simulink model "PMSM_temperature_estimation_EKF"  (R2023b)
settings: Solver=VariableStepAuto  StartTime=0.0  StopTime=10  FixedStep=dt  RelTol=1e-3  AbsTol=1e-3
values from neighbouring files (symbols this model uses):
  CF_fc = 1/(20*Ts)    (= 5)    [controller_parameters.m]
  CF_k = 1    [controller_parameters.m]
  dt = 50e-6    (= 5e-05)    [config.m]
  dt_speed_control = 0.001    [config.m]
  max_power = 50e3    (= 50000)    [config.m]
  max_torque = 220    [config.m]
  N = 6    [config.m]
  ratio_rotor = 0.75    [config.m]
  Rd_percent_rotor = ratio_rotor*100    (= 75)    [config.m]
  Rm_percent_rotor = ratio_rotor*100    (= 75)    [config.m]
  rotor_initial_temperatures = 298.15    [config.m]
  stator_initial_temperatures = [298.15;298.15;298.15]    [config.m]
  stator_thermal_mass = 100    [config.m]
  Ts = 0.01    [controller_parameters.m]
undefined symbols (not defined in the file or in its folder): cex, ch, cJ, DiscIntNeverNeededParam
libraries: fl_lib x152, nesl_utility x45, fl_ps_legacy_lib x3, sharedTrackingLibrary x1, ee_lib x1, SignalEditorBlockLib x1, simulink x1
(part 1 of 3)
Description:
  | PMSM with Thermal Model
settings Model: Creator=The MathWorks, Inc.  LastModifiedBy=block
settings SolverCC: AutoScaleAbsTol=off  AlgebraicLoopSolver=TrustRegion
settings DataIOCC: MaxDataPoints=210000  SaveFormat=Array  ReturnWorkspaceOutputsName=simOut
settings OptimizationCC: BlockReduction=off  BooleanDataType=off  LifeSpan=inf
settings DebuggingCC: SaveWithParameterizedLinksMsg=none  UnderspecifiedInitializationDetection=Classic  MergeDetectMultiDrivingBlocksExec=none  SignalResolutionControl=TryResolveAllWithWarning  UnconnectedInputMsg=warning  UnconnectedOutputMsg=warning  UnconnectedLineMsg=warning  AllowSymbolicDim=off  SFUnexpectedBacktrackingDiag=warning  SFNoUnconditionalDefaultTransitionDiag=warning  SFExecutionAtInitializationDiag=none  ArithmeticOperatorsInVariantConditions=warning
settings HardwareCC: ProdBitPerPointer=32  ProdBitPerSizeT=32  ProdBitPerPtrDiffT=32  ProdLargestAtomicFloat=None  ProdIntDivRoundTo=Undefined  ProdEndianess=Unspecified  ProdWordSize=32  ProdHWDeviceType=32-bit Generic  TargetUnknown=on
settings ModelReferenceCC: EnableRefExpFcnMdlSchedulingChecks=on  PropagateSignalLabelsOutOfModel=off
settings SFSimCC: SimUseLocalCustomCode=off  CustomCodeUndefinedFunction=UseInterfaceOnly
settings RTWCC: RTWUseLocalCustomCode=off  DLArmComputeVersion=19.05
settings CodeAppCC: StateflowObjectComments=on
settings GRTTargetCC: TargetLangStandard=C89/C90 (ANSI)
settings ConfigComp: CovMetricSettings=dw  CovSaveCumulativeToWorkspaceVar=on  CovSaveSingleToWorkspaceVar=on  CovExternalEMLEnable=off  CovSFcnEnable=off
settings SimscapeCC: SimscapeLogType=all  SimscapeLogSimulationStatistics=on  SimscapeLogName=simlog_PMSMWithThermal  SimscapeLogDecimation=10  SimscapeLogDataHistory=210000

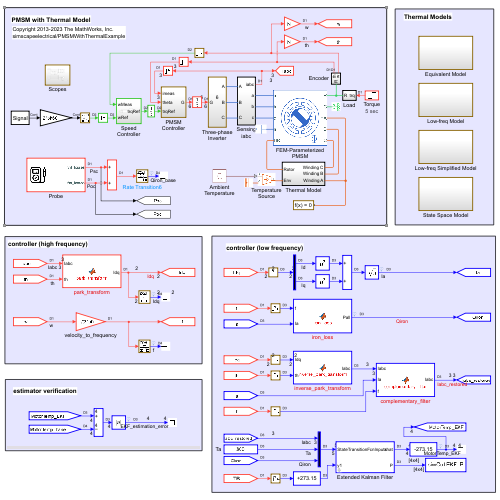
[thumbnail: Simulink's stored preview of the top-level diagram]
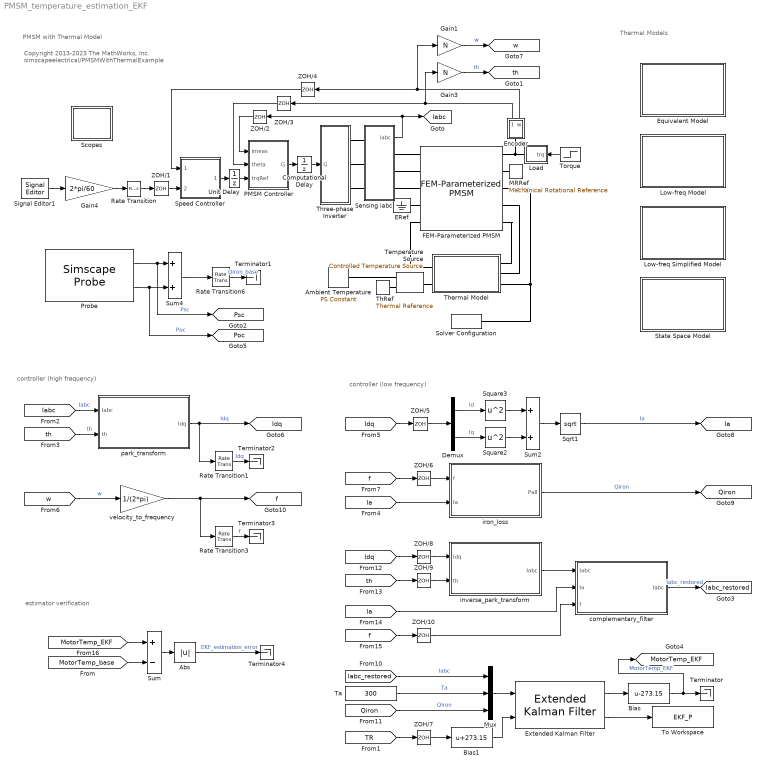
== system PMSM_temperature_estimation_EKF ==
  note: PMSM with Thermal Model
  note: controller (high frequency)
  note: controller (low frequency)
  note: Copyright 2013-2023 The MathWorks, Inc.
      | simscapeelectrical/PMSMWithThermalExample
  note: Thermal Models
  note: estimator verification
  Abs : Abs  SaturateOnIntegerOverflow=off
  Ambient Temperature : fl_lib/Physical Signals/Sources/PS Constant  constant=300
  Bias : Bias  Bias=-273.15  SaturateOnIntegerOverflow=off
  Bias1 : Bias  Bias=273.15  SaturateOnIntegerOverflow=off
  Computational Delay : UnitDelay  SampleTime=dt  HasFrameUpgradeWarning=on
  Demux : Demux  Outputs=2
  ERef : fl_lib/Electrical/Electrical Elements/Electrical Reference
  Encoder : Subsystem
  Equivalent Model : Subsystem  Tag=PublishSubsystem
  Extended Kalman Filter : sharedTrackingLibrary/Extended Kalman Filter  StateTransitionFcn=state_equation_discrete  HasStateTransitionJacobianFcn=off  HasAdditiveProcessNoise=Additive  ProcessNoise=EKF_Q  HasTimeVaryingProcessNoise=off  HasStateTransitionFcnExtraArgument=1  InitialState=EKF_x0  InitialStateCovariance=EKF_P0  MeasurementFcn1=output_equation  HasMeasurementJacobianFcn1=off  HasMeasurementEnablePort1=off  HasAdditiveMeasurementNoise1=Additive  MeasurementNoise1=EKF_R  HasTimeVaryingMeasurementNoise1=off  HasMeasurementFcnExtraArgument1=0  HasMeasurementWrapping1=off  MeasurementFcn2=myMeasurementFcn  HasMeasurementJacobianFcn2=off  HasMeasurementEnablePort2=off  HasAdditiveMeasurementNoise2=Additive  MeasurementNoise2=1  HasTimeVaryingMeasurementNoise2=off  HasMeasurementFcnExtraArgument2=0  HasMeasurementWrapping2=off  MeasurementFcn3=myMeasurementFcn  HasMeasurementJacobianFcn3=off  HasMeasurementEnablePort3=off  HasAdditiveMeasurementNoise3=Additive  MeasurementNoise3=1  HasTimeVaryingMeasurementNoise3=off  HasMeasurementFcnExtraArgument3=0  HasMeasurementWrapping3=off  MeasurementFcn4=myMeasurementFcn  HasMeasurementJacobianFcn4=off  HasMeasurementEnablePort4=off  HasAdditiveMeasurementNoise4=Additive  MeasurementNoise4=1  HasTimeVaryingMeasurementNoise4=off  HasMeasurementFcnExtraArgument4=0  HasMeasurementWrapping4=off  MeasurementFcn5=myMeasurementFcn  HasMeasurementJacobianFcn5=off  HasMeasurementEnablePort5=off  HasAdditiveMeasurementNoise5=Additive  MeasurementNoise5=1  HasTimeVaryingMeasurementNoise5=off  HasMeasurementFcnExtraArgument5=0  HasMeasurementWrapping5=off  EnableMultirate=off  StateTransitionFcnSampleTime=1  MeasurementFcn1SampleTime=1  MeasurementFcn2SampleTime=1  MeasurementFcn3SampleTime=1  MeasurementFcn4SampleTime=1  MeasurementFcn5SampleTime=1  UseCurrentEstimator=on  OutputStateCovariance=on  DataType=double  SampleTime=Ts  NumberOfMeasurements=1
  FEM-Parameterized PMSM : ee_lib/Electromechanical/Permanent Magnet/FEM-Parameterized PMSM  parameterization=1  winding_type=ee.enum.statorconnection.wye  iVec=iVec_th A  xVec=xVec_th deg  dfluxdiMatrix=dfluxdiMatrix Wb/A  dfluxdxMatrix=dfluxdxMatrix Wb/rad  calculate_torque_matrix=1  TorqueMatrix=[0, 0.3, - 0.3, 0; 0, 0, 0, 0; 0, - 0.3, 0.3, 0] N*m  idVec1=[-200.0, 0.0, 200.0] A  iqVec1=[-200.0, 0.0, 200.0] A  LdMatrix=0.0002 * ones(3, 3) H  LqMatrix=0.0002 * ones(3, 3) H  PmMatrix=0.1 * ones(3, 3) Wb  N=6  interp_method=1  Rs=Rs Ohm  Ms=Ms H  L0=0.00016 H  loss_param=ee.enum.fem_motor.ironLossesExtended.empirical  losses_oc=losses_oc W  losses_sc=losses_sc W  f_losses=f_losses Hz  Isc_losses=Isc_losses A  Inertia=0.02 kg*m^2  lam=0 N*m/(rad/s)  i_d_specify=off  i_d_priority=None  i_d=0 A  i_d_nominal_specify=off  i_d_nominal_unit=A  i_d_nominal_value=1  i_q_specify=off  i_q_priority=None  i_q=0 A  i_q_nominal_specify=off  i_q_nominal_unit=A  i_q_nominal_value=1  torque_specify=off  torque_priority=None  torque=0 N*m  torque_nominal_specify=off  torque_nominal_unit=N*m  torque_nominal_value=1  angular_velocity_specify=on  angular_velocity_priority=High  angular_velocity=0 rpm  angular_velocity_nominal_specify=off  angular_velocity_nominal_unit=rpm  angular_velocity_nominal_value=1  angular_position_specify=on  angular_position_priority=High  angular_position=0 deg  angular_position_nominal_specify=off  angular_position_nominal_unit=deg  angular_position_nominal_value=1  Tmeas=Tmeas K  alpha=alpha 1/K  alpha_flux=alpha_flux 1/K  stator_thermal_mass=stator_thermal_mass J/K  stator_initial_temperatures=stator_initial_temperatures K  rotor_thermal_mass=rotor_thermal_mass J/K  rotor_initial_temperature=rotor_initial_temperatures K  Rm_percent_rotor=Rm_percent_rotor  Rd_percent_rotor=Rm_percent_rotor  idVec=[-200, 0, 200] A  iqVec=[-200, 0, 200] A  dfluxAdiaMatrix3D=zeros(3, 3, 4) Wb/A  dfluxAdibMatrix3D=zeros(3, 3, 4) Wb/A  dfluxAdicMatrix3D=zeros(3, 3, 4) Wb/A  dfluxAdxMatrix3D=zeros(3, 3, 4) Wb/rad  TorqueMatrix3D=zeros(3, 3, 4) N*m  iaVec=[-200, 0, 200] A  ibVec=[-200, 0, 200] A  icVec=[-200, 0, 200] A  dfluxAdiaMatrix=zeros(3, 3, 3, 4) Wb/A  dfluxAdibMatrix=zeros(3, 3, 3, 4) Wb/A  dfluxAdicMatrix=zeros(3, 3, 3, 4) Wb/A  dfluxAdxMatrix=zeros(3, 3, 3, 4) Wb/rad  param_dq0=ee.enum.fem_motor.fluxTabulationOption.DQcartesian  winding_type_dq0=ee.enum.statorconnection.wye  expose_neutral_port=ee.enum.fem_motor.exposeNeutralPort.no  nPolePairs=4  parks_type=ee.enum.fem_motor.parksType.QleadsD_AphaseToDaxis  idVec2=[-200, 0, 200] A  iqVec2=[-200, 0, 200] A  magVec2=[0, 100, 200] A  betaVec2=[-180, -90, 0, 90, 180] deg  xVec2=[0, 15, 30, 45, 60, 75, 90] deg  fluxD_dq0=zeros(3, 3, 7) Wb  fluxQ_dq0=zeros(3, 3, 7) Wb  fluxA_dq0=zeros(3, 3, 7) Wb  Torque_dq0=ones(3, 3, 7) N*m  fluxD_IBX=zeros(3, 5, 7) Wb  fluxQ_IBX=zeros(3, 5, 7) Wb  fluxA_IBX=zeros(3, 5, 7) Wb  Torque_IBX=zeros(3, 5, 7) N*m  rotorLossCoeff_k_h_DQ=zeros(3, 3) W/Hz  rotorLossCoeff_k_J_DQ=zeros(3, 3) W/Hz^2  rotorLossCoeff_k_ex_DQ=zeros(3, 3) W/Hz^(3/2)  rotorLossCoeff_k_h_IB=zeros(3, 5) W/Hz  rotorLossCoeff_k_J_IB=zeros(3, 5) W/Hz^2  rotorLossCoeff_k_ex_IB=zeros(3, 5) W/Hz^(3/2)  statorLossCoeff_k_h_DQ=zeros(3, 3) W/Hz  statorLossCoeff_k_J_DQ=zeros(3, 3) W/Hz^2  statorLossCoeff_k_ex_DQ=zeros(3, 3) W/Hz^(3/2)  statorLossCoeff_k_h_IB=zeros(3, 5) W/Hz  statorLossCoeff_k_J_IB=zeros(3, 5) W/Hz^2  statorLossCoeff_k_ex_IB=zeros(3, 5) W/Hz^(3/2)  wVec=[1000, 2000] rpm  rotorLossTable_DQ=zeros(3, 3, 2) W  rotorLossTable_IB=zeros(3, 5, 2) W  statorLossTable_DQ=zeros(3, 3, 2) W  statorLossTable_IB=zeros(3, 5, 2) W  electrical_torque_before_iron_losses_specify=off  electrical_torque_before_iron_losses_priority=None  electrical_torque_before_iron_losses=0 N*m  electrical_torque_before_iron_losses_nominal_specify=off  electrical_torque_before_iron_losses_nominal_unit=N*m  electrical_torque_before_iron_losses_nominal_value=1  Qrotor_specify=off  Qrotor_priority=None  Qrotor=0 J/s  Qrotor_nominal_specify=off  Qrotor_nominal_unit=J/s  Qrotor_nominal_value=1  Qstator_specify=off  Qstator_priority=None  Qstator=0 J/s  Qstator_nominal_specify=off  Qstator_nominal_unit=J/s  Qstator_nominal_value=1
      settings: InternalSimscapePortConfiguration="{\"Bottom\":[],\"Left\":[{\"id\":\"a\",\"label\":\"a\",\"type\":\"foundation.electrical.electrical\"},{\"id\":\"b\",\"label\":\"b\",\"type\":\"foundation.electrical.electrical\"},{\"id\":\"c\",\"label\":\"c\",\"type\":\"foundation.electrical.electrical\"},{\"id\":\"n\",\"label\":\"n\",\"type\":\"foundation.electrical.electrical\"},{\"id\":\"HR\",\"label\":\"HR\",\"type\":\"foundation.thermal.thermal\"}],\"Right\":[{\"id\":\"R\",\"label\":\"R\",\"type\":\"foundation.mechanical.rotational.rotational\"},{\"id\":\"C\",\"label\":\"C\",\"type\":\"foundation.mechanical.rotational.rotational\"},{\"id\":\"HA\",\"label\":\"HA\",\"type\":\"foundation.thermal.thermal\"},{\"id\":\"HB\",\"label\":\"HB\",\"type\":\"foundation.thermal.thermal\"},{\"id\":\"HC\",\"label\":\"HC\",\"type\":\"foundation.thermal.thermal\"}],\"Top\":[]}"
  Gain1 : Gain  Gain=N
  Gain3 : Gain  Gain=N
  Gain4 : Gain  Gain=2*pi/60
  Load : Subsystem
  Low-freq Model : Subsystem  Tag=PublishSubsystem
  Low-freq Simplified Model : Subsystem  Tag=PublishSubsystem
  MRRef : fl_lib/Mechanical/Rotational Elements/Mechanical Rotational Reference
  Mux : Mux  Inputs=3
  PMSM Controller : Subsystem
  Probe : SimscapeProbe  BoundBlock=1888  Variables={Vd_losses, Vm_losses}
  Rate Transition : RateTransition
  Rate Transition1 : RateTransition  OutPortSampleTime=dt_display
  Rate Transition3 : RateTransition  OutPortSampleTime=dt_display
  Rate Transition6 : RateTransition  OutPortSampleTime=dt_display
  Scopes : Subsystem
  Sensing iabc : Subsystem
  Signal Editor1 : SignalEditorBlockLib/Signal Editor  FileName=target_speed.mat  ActiveScenario=Scenario  ActiveSignal=Signal  IsBus=off  OutputBusObjectStr=Bus: BusObject  SampleTime=0  Interpolate=off  ZeroCross=off  OutputAfterFinalValue=Setting to zero  Unit=inherit  PreserveSignalName=on  ApplySigPropsToAllScenarios=on  ApplySigPropsToAllSignals=off
  Solver Configuration : nesl_utility/Solver Configuration  PhysicalDomain=network_engine_domain  SubClassName=solver  LeftPortType=input  RightPortType=generic  Tones=[]  Harmonics=[]  SimulateNoise=off  Profile=off  UseLocalSampling=off  EnableSwitchedLinearOptims=on  FrequencyDomain=off  UseCCode=off  RelTol=0.001  AbsTol=1e-06  MinStep=1e-09  ToWorkspace=off  RevertToSquareIcSolve=off  NumHomotopyIterations=100  PhasorMode=off  PhasorModeNumHarmonics=1  ConsistencySolver=NEWTON_FTOL  IndexReductionMethod=DerivativeReplacement  DoDC=off  ResidualTolerance=1e-9  ConsistencyTolSource=GLOBAL  ConsistencyAbsTol=0.001  ConsistencyRelTol=0.001  ConsistencyTolFactor=0.001  UseLocalSolver=on  LocalSolverChoice=NE_BACKWARD_EULER_ADVANCER  ResolveIndetEquations=on  FunctionEvalNumThread=1  LocalSolverSampleTime=dt  DoFixedCost=on  MaxNonlinIter=3  MaxModeIter=2  ComputeImpulses=off  ImpulseIterations=2  LinearAlgebra=auto  LinearAlgebraNumThread=0  EquationFormulation=NE_TIME_EF  DelaysMemoryBudget=1024  AutomaticFiltering=on  FilteringTimeConstant=0.001  PartitionStorageMethod=AS_NEEDED  PartitionMemoryBudget=1024  PartitionMethod=FAST  MultibodyUseLocalSolver=off  MultibodyLocalSolverChoice=ODE1  MultibodyLocalSolverSampleTime=0.001
  Speed Controller : Subsystem
  Sqrt1 : Sqrt
  Square2 : Math  Operator=square
  Square3 : Math  Operator=square
  State Space Model : Subsystem  Tag=PublishSubsystem
  Sum : Sum  Inputs=+-
  Sum2 : Sum
  Sum4 : Sum
  Ta : Constant  Value=300  SampleTime=Ts
  Temperature Source : fl_lib/Thermal/Thermal Sources/Controlled Temperature Source
  Terminator{,1..4} (5 alike) : Terminator
  ThRef : fl_lib/Thermal/Thermal Elements/Thermal Reference
  Thermal Model : Subsystem  Tag=PublishSubsystem
  Three-phase Inverter : Subsystem  VariantControl=Variant
  To Workspace : ToWorkspace  VariableName=EKF_P  SampleTime=-1
      settings: MaxDataPoints=1
  Torque : Step  Time=5  After=100  SampleTime=dt
      settings: AttributesFormatString=%<Time> sec
  Unit Delay : UnitDelay  SampleTime=dt_speed_control  HasFrameUpgradeWarning=on
  ZOH/1 : ZeroOrderHold  SampleTime=dt_speed_control
  ZOH/{5..10} (6 alike) : ZeroOrderHold  SampleTime=Ts
  ZOH/2 : ZeroOrderHold  SampleTime=dt
  ZOH/3 : ZeroOrderHold  SampleTime=dt
  ZOH/4 : ZeroOrderHold  SampleTime=dt_speed_control
  complementary_filter : MATLAB Function  TreatAsAtomicUnit=on
  inverse_park_transform : MATLAB Function  TreatAsAtomicUnit=on
  iron_loss : MATLAB Function  TreatAsAtomicUnit=on
  park_transform : MATLAB Function  TreatAsAtomicUnit=on
  velocity_to_frequency : Gain  Gain=1/(2*pi)
  tag scope: Ia=global, Iabc=global, Iabc_restored=global, Idq=global, MotorTemp_EKF=global, Poc=global, Psc=global, Qiron=global, f=global, th=global, w=global
  wires:
  Encoder/2(w) -> ZOH/4/1, Gain1/1
  ZOH/4/1 -> Speed Controller/1(wMeas)
  Speed Controller/1(trqRef) -> Unit Delay/1
  ZOH/1/1 -> Speed Controller/2(wRef)
  ZOH/3/1 -> PMSM Controller/2(theta)
  ZOH/2/1 -> PMSM Controller/1(imeas)
  PMSM Controller/1(G) -> Computational Delay/1
  Unit Delay/1 -> PMSM Controller/3(trqRef)
  Encoder/1(th) -> ZOH/3/1, Gain3/1
  Computational Delay/1 -> Three-phase Inverter/1(G)
  Sensing iabc/1(iabc) -> [Iabc], ZOH/2/1
  Torque/1 -> Load/1(trq)
  Rate Transition/1 -> ZOH/1/1
  Signal Editor1/1 -> Gain4/1
  [Iabc] -> park_transform/1(Iabc)  "Iabc"
  [th] -> park_transform/2(th)  "th"
  Probe/1 -> [Psc], Sum4/1  "Psc"
  Gain1/1 -> [w]  "w"
  Gain3/1 -> [th]  "th"
  park_transform/1(Idq) -> [Idq], Rate Transition1/1  "Idq"
  Gain4/1 -> Rate Transition/1
  ZOH/5/1 -> Demux/1
  Demux/2 -> Square2/1  "Iq"
  Demux/1 -> Square3/1  "Id"
  Square3/1 -> Sum2/1
  Square2/1 -> Sum2/2
  Sum2/1 -> Sqrt1/1
  Sqrt1/1 -> [Ia]  "Ia"
  iron_loss/1(Pall) -> [Qiron]  "Qiron"
  [f] -> ZOH/6/1
  Rate Transition6/1 -> Terminator1/1  "Qiron_base"
  Rate Transition1/1 -> Terminator2/1  "Idq"
  [Idq] -> ZOH/5/1
  [w] -> velocity_to_frequency/1  "w"
  velocity_to_frequency/1 -> [f], Rate Transition3/1
  Rate Transition3/1 -> Terminator3/1  "f"
  Sum4/1 -> Rate Transition6/1
  ZOH/6/1 -> iron_loss/1(f)
  [Ia] -> iron_loss/2(Ia)
  Probe/2 -> [Poc], Sum4/2  "Poc"
  Ta/1 -> Mux/2  "Ta"
  [Iabc_restored] -> Mux/1  "Iabc"
  [Qiron] -> Mux/3  "Qiron"
  [TR] -> ZOH/7/1
  Mux/1 -> Extended Kalman Filter/1
  ZOH/7/1 -> Bias1/1
  Bias/1 -> [MotorTemp_EKF], Terminator/1  "MotorTemp_EKF"
  Extended Kalman Filter/1 -> Bias/1
  Bias1/1 -> Extended Kalman Filter/2
  [Idq] -> ZOH/8/1
  ZOH/8/1 -> inverse_park_transform/1(Idq)
  ZOH/9/1 -> inverse_park_transform/2(th)
  [th] -> ZOH/9/1
  inverse_park_transform/1(Iabc) -> complementary_filter/1("Iabc ")
  [Ia] -> complementary_filter/2(Ia)
  [f] -> ZOH/10/1
  ZOH/10/1 -> complementary_filter/3(f)
  complementary_filter/1(Iabc) -> [Iabc_restored]  "Iabc_restored"
  Extended Kalman Filter/2 -> To Workspace/1
  [MotorTemp_EKF] -> Sum/1
  [MotorTemp_base] -> Sum/2
  Abs/1 -> Terminator4/1  "EKF_estimation_error"
  Sum/1 -> Abs/1
  connections:
  FEM-Parameterized PMSM/LConn4 -- ERef/LConn1
  FEM-Parameterized PMSM/RConn4 -- Thermal Model/RConn2
  FEM-Parameterized PMSM/RConn5 -- Thermal Model/RConn1
  FEM-Parameterized PMSM/RConn3 -- Solver Configuration/RConn1 -- Thermal Model/RConn3
  MRRef/LConn1 -- FEM-Parameterized PMSM/RConn2
  FEM-Parameterized PMSM/RConn1 -- Encoder/LConn1 -- Load/RConn1
  Three-phase Inverter/RConn1 -- Sensing iabc/LConn1
  FEM-Parameterized PMSM/LConn1 -- Sensing iabc/RConn1
  Three-phase Inverter/RConn2 -- Sensing iabc/LConn2
  FEM-Parameterized PMSM/LConn2 -- Sensing iabc/RConn2
  Three-phase Inverter/RConn3 -- Sensing iabc/LConn3
  FEM-Parameterized PMSM/LConn3 -- Sensing iabc/RConn3
  Ambient Temperature/RConn1 -- Temperature Source/RConn1
  ThRef/LConn1 -- Temperature Source/RConn2
  Temperature Source/LConn1 -- Thermal Model/LConn2
  Thermal Model/LConn1 -- FEM-Parameterized PMSM/LConn5

== system PMSM_temperature_estimation_EKF/Encoder ==
  MRRef : fl_lib/Mechanical/Rotational Elements/Mechanical Rotational Reference
  Motion Sensor : fl_lib/Mechanical/Mechanical Sensors/Ideal Rotational Motion Sensor  reference=foundation.enum.MeasurementReference.difference  acceleration_port=false  velocity_port=true  position_port=true  wrap_angle=simscape.enum.onoff.off  offset=0 deg
  PS-Simulink Converter : nesl_utility/PS-Simulink Converter  PhysicalDomain=network_engine_domain  SubClassName=ps_output  LeftPortType=input  RightPortType=output  PseudoPeriodic=off  Frequencies=[]  VectorFormat=1-D array  Unit=rad/s  AffineConversion=off
  PS-Simulink Converter1 : nesl_utility/PS-Simulink Converter  PhysicalDomain=network_engine_domain  SubClassName=ps_output  LeftPortType=input  RightPortType=output  PseudoPeriodic=off  Frequencies=[]  VectorFormat=1-D array  Unit=rad  AffineConversion=off
  R : PMIOPort  Side=Left
  th : Outport  VectorParamsAs1DForOutWhenUnconnected=off
  w : Outport  Port=2  VectorParamsAs1DForOutWhenUnconnected=off
  tag scope: wMotor=global
  wires:
  PS-Simulink Converter1/1 -> th/1
  PS-Simulink Converter/1 -> w/1, [wMotor]
  connections:
  Motion Sensor/RConn2 -- PS-Simulink Converter/LConn1
  Motion Sensor/RConn3 -- PS-Simulink Converter1/LConn1
  MRRef/LConn1 -- Motion Sensor/RConn1
  Motion Sensor/LConn1 -- R/RConn1

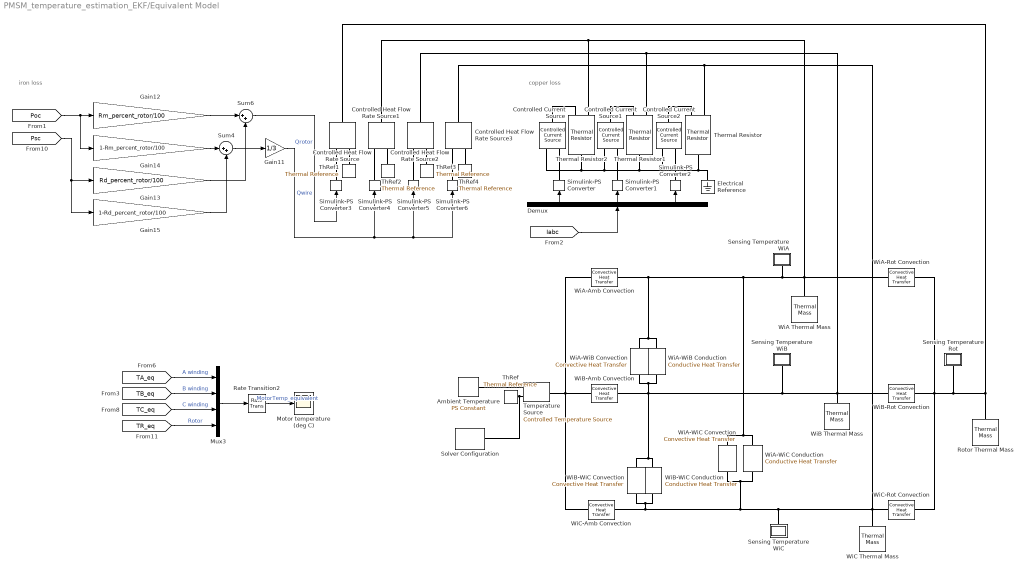
== system PMSM_temperature_estimation_EKF/Equivalent Model ==
  note: iron loss
  note: copper loss
  Ambient Temperature : fl_lib/Physical Signals/Sources/PS Constant  constant=300
  Controlled Current Source : fl_lib/Electrical/Electrical Sources/Controlled Current Source
  Controlled Current Source1 : fl_lib/Electrical/Electrical Sources/Controlled Current Source
  Controlled Current Source2 : fl_lib/Electrical/Electrical Sources/Controlled Current Source
  Controlled Heat Flow Rate Source{,1..3} (4 alike) : fl_lib/Thermal/Thermal Sources/Controlled Heat Flow Rate Source
  Demux : Demux  Outputs=3
  Electrical Reference : fl_lib/Electrical/Electrical Elements/Electrical Reference
  Gain11 : Gain  Gain=1/3
  Gain12 : Gain  Gain=Rm_percent_rotor/100
  Gain13 : Gain  Gain=Rd_percent_rotor/100
  Gain14 : Gain  Gain=1-Rm_percent_rotor/100
  Gain15 : Gain  Gain=1-Rd_percent_rotor/100
  Motor temperature (deg C) : Scope
  Mux3 : Mux
  Rate Transition2 : RateTransition  OutPortSampleTime=dt_display
  Rotor Thermal Mass : fl_lib/Thermal/Thermal Elements/Thermal Mass  mass_type=foundation.enum.constant_variable.constant  mass=1 kg  sp_heat=rotor_thermal_mass J/(K*kg)  mass_min=1e-6 kg  num_ports=foundation.enum.numPorts2.one  m_specify=off  m_priority=High  m=1 kg  m_nominal_specify=off  m_nominal_unit=kg  m_nominal_value=1  T_specify=on  T_priority=High  T=rotor_initial_temperatures K  T_nominal_specify=off  T_nominal_unit=K  T_nominal_value=1  Q_specify=off  Q_priority=High  Q=0 W  Q_nominal_specify=off  Q_nominal_unit=W  Q_nominal_value=1
  Sensing Temperature Rot : Subsystem
      mask Display: disp('TR')
  Sensing Temperature WiA : Subsystem
      mask Display: disp('TA')
  Sensing Temperature WiB : Subsystem
      mask Display: disp('TB')
  Sensing Temperature WiC : Subsystem
      mask Display: disp('TC')
  Simulink-PS Converter : nesl_utility/Simulink-PS Converter  PhysicalDomain=network_engine_domain  SubClassName=ps_input  LeftPortType=input  RightPortType=output  PseudoPeriodic=off  Frequencies=[]  NoiseDistribution=none  NoiseParameters=[]  Unit=A  AffineConversion=off  FilteringAndDerivatives=provide  SimscapeFilterOrder=1  InputFilterTimeConstant=0.001  UdotUserProvided=0
  Simulink-PS Converter1 : nesl_utility/Simulink-PS Converter  PhysicalDomain=network_engine_domain  SubClassName=ps_input  LeftPortType=input  RightPortType=output  PseudoPeriodic=off  Frequencies=[]  NoiseDistribution=none  NoiseParameters=[]  Unit=A  AffineConversion=off  FilteringAndDerivatives=provide  SimscapeFilterOrder=1  InputFilterTimeConstant=0.001  UdotUserProvided=0
  Simulink-PS Converter2 : nesl_utility/Simulink-PS Converter  PhysicalDomain=network_engine_domain  SubClassName=ps_input  LeftPortType=input  RightPortType=output  PseudoPeriodic=off  Frequencies=[]  NoiseDistribution=none  NoiseParameters=[]  Unit=A  AffineConversion=off  FilteringAndDerivatives=provide  SimscapeFilterOrder=1  InputFilterTimeConstant=0.001  UdotUserProvided=0
  Simulink-PS Converter{3..6} (4 alike) : nesl_utility/Simulink-PS Converter  PhysicalDomain=network_engine_domain  SubClassName=ps_input  LeftPortType=input  RightPortType=output  PseudoPeriodic=off  Frequencies=[]  NoiseDistribution=none  NoiseParameters=[]  Unit=J/s  AffineConversion=off  FilteringAndDerivatives=provide  SimscapeFilterOrder=1  InputFilterTimeConstant=0.001  UdotUserProvided=0
  Solver Configuration : nesl_utility/Solver Configuration  PhysicalDomain=network_engine_domain  SubClassName=solver  LeftPortType=input  RightPortType=generic  Tones=[]  Harmonics=[]  SimulateNoise=off  Profile=off  UseLocalSampling=off  EnableSwitchedLinearOptims=on  FrequencyDomain=off  UseCCode=off  RelTol=0.001  AbsTol=0.001  MinStep=1e-09  ToWorkspace=off  RevertToSquareIcSolve=off  NumHomotopyIterations=100  PhasorMode=off  PhasorModeNumHarmonics=1  ConsistencySolver=NEWTON_XTOL_AFTER_FTOL  IndexReductionMethod=DerivativeReplacement  DoDC=off  ResidualTolerance=1e-09  ConsistencyTolSource=GLOBAL  ConsistencyAbsTol=0.001  ConsistencyRelTol=0.001  ConsistencyTolFactor=0.001  UseLocalSolver=off  LocalSolverChoice=NE_BACKWARD_EULER_ADVANCER  ResolveIndetEquations=on  FunctionEvalNumThread=1  LocalSolverSampleTime=0.001  DoFixedCost=off  MaxNonlinIter=3  MaxModeIter=2  ComputeImpulses=off  ImpulseIterations=2  LinearAlgebra=auto  LinearAlgebraNumThread=0  EquationFormulation=NE_TIME_EF  DelaysMemoryBudget=1024  AutomaticFiltering=on  FilteringTimeConstant=0.001  PartitionStorageMethod=AS_NEEDED  PartitionMemoryBudget=1024  PartitionMethod=ROBUST  MultibodyUseLocalSolver=off  MultibodyLocalSolverChoice=ODE1  MultibodyLocalSolverSampleTime=0.001
  Sum4 : Sum  Inputs=|++
  Sum6 : Sum  Inputs=|++
  Temperature Source : fl_lib/Thermal/Thermal Sources/Controlled Temperature Source
  ThRef{,1..4} (5 alike) : fl_lib/Thermal/Thermal Elements/Thermal Reference
  Thermal Resistor : fl_lib/Electrical/Electrical Elements/Thermal Resistor  R0=Rs Ohm  T0=Tmeas K  alpha=alpha 1/K  tc=0.1 s  K_d=1e-3 W/K  T_specify=on  T_priority=High  T=stator_initial_temperatures(3) K  T_nominal_specify=off  T_nominal_unit=K  T_nominal_value=1
      settings: InternalSimscapePortConfiguration="{\"Bottom\":[],\"Left\":[{\"id\":\"H\",\"label\":\"H\",\"type\":\"foundation.thermal.thermal\"},{\"id\":\"p\",\"label\":\"+\",\"type\":\"foundation.electrical.electrical\"}],\"Right\":[{\"id\":\"n\",\"label\":\"-\",\"type\":\"foundation.electrical.electrical\"}],\"Top\":[]}"
  Thermal Resistor1 : fl_lib/Electrical/Electrical Elements/Thermal Resistor  R0=Rs Ohm  T0=Tmeas K  alpha=alpha 1/K  tc=0.1 s  K_d=1e-3 W/K  T_specify=on  T_priority=High  T=stator_initial_temperatures(2) K  T_nominal_specify=off  T_nominal_unit=K  T_nominal_value=1
      settings: InternalSimscapePortConfiguration="{\"Bottom\":[],\"Left\":[{\"id\":\"H\",\"label\":\"H\",\"type\":\"foundation.thermal.thermal\"},{\"id\":\"p\",\"label\":\"+\",\"type\":\"foundation.electrical.electrical\"}],\"Right\":[{\"id\":\"n\",\"label\":\"-\",\"type\":\"foundation.electrical.electrical\"}],\"Top\":[]}"
  Thermal Resistor2 : fl_lib/Electrical/Electrical Elements/Thermal Resistor  R0=Rs Ohm  T0=Tmeas K  alpha=alpha 1/K  tc=0.1 s  K_d=1e-3 W/K  T_specify=on  T_priority=High  T=stator_initial_temperatures(1) K  T_nominal_specify=off  T_nominal_unit=K  T_nominal_value=1
      settings: InternalSimscapePortConfiguration="{\"Bottom\":[],\"Left\":[{\"id\":\"H\",\"label\":\"H\",\"type\":\"foundation.thermal.thermal\"},{\"id\":\"p\",\"label\":\"+\",\"type\":\"foundation.electrical.electrical\"}],\"Right\":[{\"id\":\"n\",\"label\":\"-\",\"type\":\"foundation.electrical.electrical\"}],\"Top\":[]}"
  WiA Thermal Mass : fl_lib/Thermal/Thermal Elements/Thermal Mass  mass_type=foundation.enum.constant_variable.constant  mass=1 kg  sp_heat=stator_thermal_mass J/(K*kg)  mass_min=1e-6 kg  num_ports=foundation.enum.numPorts2.one  m_specify=off  m_priority=High  m=1 kg  m_nominal_specify=off  m_nominal_unit=kg  m_nominal_value=1  T_specify=on  T_priority=High  T=stator_initial_temperatures(1) K  T_nominal_specify=off  T_nominal_unit=K  T_nominal_value=1  Q_specify=off  Q_priority=High  Q=0 W  Q_nominal_specify=off  Q_nominal_unit=W  Q_nominal_value=1
  WiA-Amb Convection : fl_lib/Thermal/Thermal Elements/Convective Heat Transfer  thermal_type=foundation.enum.constant_variable.constant  area=0.1 m^2  heat_tr_coeff=20 W/(m^2 * K)  min_heat_tr_coeff=1e-3 W/(K*m^2)  T_specify=off  T_priority=None  T=0 K  T_nominal_specify=off  T_nominal_unit=K  T_nominal_value=1  Q_specify=off  Q_priority=None  Q=0 J/s  Q_nominal_specify=off  Q_nominal_unit=J/s  Q_nominal_value=1
  WiA-Rot Convection : fl_lib/Thermal/Thermal Elements/Convective Heat Transfer  thermal_type=foundation.enum.constant_variable.constant  area=0.02 m^2  heat_tr_coeff=200 W/(m^2 * K)  min_heat_tr_coeff=1e-3 W/(K*m^2)  T_specify=off  T_priority=None  T=0 K  T_nominal_specify=off  T_nominal_unit=K  T_nominal_value=1  Q_specify=off  Q_priority=None  Q=0 J/s  Q_nominal_specify=off  Q_nominal_unit=J/s  Q_nominal_value=1
  WiA-WiB Conduction : fl_lib/Thermal/Thermal Elements/Conductive Heat Transfer  thermal_type=foundation.enum.ConstantVariableTabulated.Constant  wall_geometry=foundation.enum.ConductionWallGeometry.Planar  area=0.002 m^2  thickness=0.1 m  d_in=0.05 m  d_out=0.1 m  L=1 m  th_cond_min=10 W/(K*m)  th_cond=80 W/(m*K)  th_cond_TLU=[413, 401, 392, 383, 371, 357, 342] W/(K*m)  temp_TLU=[200, 273, 400, 600, 800, 1000, 1200] K  T_specify=off  T_priority=None  T=0 K  T_nominal_specify=off  T_nominal_unit=K  T_nominal_value=1  Q_specify=off  Q_priority=None  Q=0 J/s  Q_nominal_specify=off  Q_nominal_unit=J/s  Q_nominal_value=1
  WiA-WiB Convection : fl_lib/Thermal/Thermal Elements/Convective Heat Transfer  thermal_type=foundation.enum.constant_variable.constant  area=0.004 m^2  heat_tr_coeff=200 W/(m^2 * K)  min_heat_tr_coeff=1e-3 W/(K*m^2)  T_specify=off  T_priority=None  T=0 K  T_nominal_specify=off  T_nominal_unit=K  T_nominal_value=1  Q_specify=off  Q_priority=None  Q=0 J/s  Q_nominal_specify=off  Q_nominal_unit=J/s  Q_nominal_value=1
  WiA-WiC Conduction : fl_lib/Thermal/Thermal Elements/Conductive Heat Transfer  thermal_type=foundation.enum.ConstantVariableTabulated.Constant  wall_geometry=foundation.enum.ConductionWallGeometry.Planar  area=0.002 m^2  thickness=0.1 m  d_in=0.05 m  d_out=0.1 m  L=1 m  th_cond_min=10 W/(K*m)  th_cond=80 W/(m*K)  th_cond_TLU=[413, 401, 392, 383, 371, 357, 342] W/(K*m)  temp_TLU=[200, 273, 400, 600, 800, 1000, 1200] K  T_specify=off  T_priority=None  T=0 K  T_nominal_specify=off  T_nominal_unit=K  T_nominal_value=1  Q_specify=off  Q_priority=None  Q=0 J/s  Q_nominal_specify=off  Q_nominal_unit=J/s  Q_nominal_value=1
  WiA-WiC Convection : fl_lib/Thermal/Thermal Elements/Convective Heat Transfer  thermal_type=foundation.enum.constant_variable.constant  area=0.004 m^2  heat_tr_coeff=200 W/(m^2 * K)  min_heat_tr_coeff=1e-3 W/(K*m^2)  T_specify=off  T_priority=None  T=0 K  T_nominal_specify=off  T_nominal_unit=K  T_nominal_value=1  Q_specify=off  Q_priority=None  Q=0 J/s  Q_nominal_specify=off  Q_nominal_unit=J/s  Q_nominal_value=1
  WiB Thermal Mass : fl_lib/Thermal/Thermal Elements/Thermal Mass  mass_type=foundation.enum.constant_variable.constant  mass=1 kg  sp_heat=stator_thermal_mass J/(K*kg)  mass_min=1e-6 kg  num_ports=foundation.enum.numPorts2.one  m_specify=off  m_priority=High  m=1 kg  m_nominal_specify=off  m_nominal_unit=kg  m_nominal_value=1  T_specify=on  T_priority=High  T=stator_initial_temperatures(2) K  T_nominal_specify=off  T_nominal_unit=K  T_nominal_value=1  Q_specify=off  Q_priority=High  Q=0 W  Q_nominal_specify=off  Q_nominal_unit=W  Q_nominal_value=1
  WiB-Amb Convection : fl_lib/Thermal/Thermal Elements/Convective Heat Transfer  thermal_type=foundation.enum.constant_variable.constant  area=0.1 m^2  heat_tr_coeff=20 W/(m^2 * K)  min_heat_tr_coeff=1e-3 W/(K*m^2)  T_specify=off  T_priority=None  T=0 K  T_nominal_specify=off  T_nominal_unit=K  T_nominal_value=1  Q_specify=off  Q_priority=None  Q=0 J/s  Q_nominal_specify=off  Q_nominal_unit=J/s  Q_nominal_value=1
  WiB-Rot Convection : fl_lib/Thermal/Thermal Elements/Convective Heat Transfer  thermal_type=foundation.enum.constant_variable.constant  area=0.02 m^2  heat_tr_coeff=200 W/(m^2 * K)  min_heat_tr_coeff=1e-3 W/(K*m^2)  T_specify=off  T_priority=None  T=0 K  T_nominal_specify=off  T_nominal_unit=K  T_nominal_value=1  Q_specify=off  Q_priority=None  Q=0 J/s  Q_nominal_specify=off  Q_nominal_unit=J/s  Q_nominal_value=1
  WiB-WiC Conduction : fl_lib/Thermal/Thermal Elements/Conductive Heat Transfer  thermal_type=foundation.enum.ConstantVariableTabulated.Constant  wall_geometry=foundation.enum.ConductionWallGeometry.Planar  area=0.002 m^2  thickness=0.1 m  d_in=0.05 m  d_out=0.1 m  L=1 m  th_cond_min=10 W/(K*m)  th_cond=80 W/(m*K)  th_cond_TLU=[413, 401, 392, 383, 371, 357, 342] W/(K*m)  temp_TLU=[200, 273, 400, 600, 800, 1000, 1200] K  T_specify=off  T_priority=None  T=0 K  T_nominal_specify=off  T_nominal_unit=K  T_nominal_value=1  Q_specify=off  Q_priority=None  Q=0 J/s  Q_nominal_specify=off  Q_nominal_unit=J/s  Q_nominal_value=1
  WiB-WiC Convection : fl_lib/Thermal/Thermal Elements/Convective Heat Transfer  thermal_type=foundation.enum.constant_variable.constant  area=0.004 m^2  heat_tr_coeff=200 W/(m^2 * K)  min_heat_tr_coeff=1e-3 W/(K*m^2)  T_specify=off  T_priority=None  T=0 K  T_nominal_specify=off  T_nominal_unit=K  T_nominal_value=1  Q_specify=off  Q_priority=None  Q=0 J/s  Q_nominal_specify=off  Q_nominal_unit=J/s  Q_nominal_value=1
  WiC Thermal Mass : fl_lib/Thermal/Thermal Elements/Thermal Mass  mass_type=foundation.enum.constant_variable.constant  mass=1 kg  sp_heat=stator_thermal_mass J/(K*kg)  mass_min=1e-6 kg  num_ports=foundation.enum.numPorts2.one  m_specify=off  m_priority=High  m=1 kg  m_nominal_specify=off  m_nominal_unit=kg  m_nominal_value=1  T_specify=on  T_priority=High  T=stator_initial_temperatures(3) K  T_nominal_specify=off  T_nominal_unit=K  T_nominal_value=1  Q_specify=off  Q_priority=High  Q=0 W  Q_nominal_specify=off  Q_nominal_unit=W  Q_nominal_value=1
  WiC-Amb Convection : fl_lib/Thermal/Thermal Elements/Convective Heat Transfer  thermal_type=foundation.enum.constant_variable.constant  area=0.1 m^2  heat_tr_coeff=20 W/(m^2 * K)  min_heat_tr_coeff=1e-3 W/(K*m^2)  T_specify=off  T_priority=None  T=0 K  T_nominal_specify=off  T_nominal_unit=K  T_nominal_value=1  Q_specify=off  Q_priority=None  Q=0 J/s  Q_nominal_specify=off  Q_nominal_unit=J/s  Q_nominal_value=1
  WiC-Rot Convection : fl_lib/Thermal/Thermal Elements/Convective Heat Transfer  thermal_type=foundation.enum.constant_variable.constant  area=0.02 m^2  heat_tr_coeff=200 W/(m^2 * K)  min_heat_tr_coeff=1e-3 W/(K*m^2)  T_specify=off  T_priority=None  T=0 K  T_nominal_specify=off  T_nominal_unit=K  T_nominal_value=1  Q_specify=off  Q_priority=None  Q=0 J/s  Q_nominal_specify=off  Q_nominal_unit=J/s  Q_nominal_value=1
  wires:
  Rate Transition2/1 -> Motor temperature (deg C)/1  "MotorTemp_equivalent"
  [TA_eq] -> Mux3/1  "A winding"
  [TR_eq] -> Mux3/4  "Rotor"
  [TC_eq] -> Mux3/3  "C winding"
  [TB_eq] -> Mux3/2  "B winding"
  Mux3/1 -> Rate Transition2/1
  Gain14/1 -> Sum4/1
  [Psc] -> Gain15/1, Gain13/1
  Gain13/1 -> Sum6/2
  Gain12/1 -> Sum6/1
  Gain11/1 -> Simulink-PS Converter4/1, Simulink-PS Converter6/1, Simulink-PS Converter5/1  "Qwire"
  Sum6/1 -> Simulink-PS Converter3/1  "Qrotor"
  Gain15/1 -> Sum4/2
  Sum4/1 -> Gain11/1
  Demux/1 -> Simulink-PS Converter/1
  Demux/2 -> Simulink-PS Converter1/1
  Demux/3 -> Simulink-PS Converter2/1
  [Iabc] -> Demux/1
  [Poc] -> Gain14/1, Gain12/1
  connections:
  WiA-Rot Convection/RConn1 -- Sensing Temperature WiA/LConn1 -- WiA-WiC Convection/RConn1 -- WiA-WiC Conduction/RConn1 -- WiA-WiB Convection/LConn1 -- WiA-WiB Conduction/LConn1 -- WiA-Amb Convection/LConn1 -- Controlled Heat Flow Rate Source1/LConn1 -- Thermal Resistor2/LConn1 -- WiA Thermal Mass/LConn1
  Sensing Temperature Rot/LConn1 -- Controlled Heat Flow Rate Source/LConn1 -- Rotor Thermal Mass/LConn1 -- WiB-Rot Convection/LConn1 -- WiA-Rot Convection/LConn1 -- WiC-Rot Convection/LConn1
  WiA-WiB Convection/RConn1 -- WiA-WiB Conduction/RConn1 -- WiB-Rot Convection/RConn1 -- Controlled Heat Flow Rate Source2/LConn1 -- Thermal Resistor1/LConn1 -- WiB Thermal Mass/LConn1 -- Sensing Temperature WiB/LConn1 -- WiB-Amb Convection/LConn1 -- WiB-WiC Convection/LConn1 -- WiB-WiC Conduction/LConn1
  WiC-Rot Convection/RConn1 -- WiB-WiC Conduction/RConn1 -- WiB-WiC Convection/RConn1 -- WiC-Amb Convection/LConn1 -- WiA-WiC Convection/LConn1 -- WiA-WiC Conduction/LConn1 -- Sensing Temperature WiC/LConn1 -- Controlled Heat Flow Rate Source3/LConn1 -- Thermal Resistor/LConn1 -- WiC Thermal Mass/LConn1
  WiA-Amb Convection/RConn1 -- Temperature Source/LConn1 -- WiC-Amb Convection/RConn1 -- WiB-Amb Convection/RConn1
  Ambient Temperature/RConn1 -- Temperature Source/RConn1
  ThRef/LConn1 -- Solver Configuration/RConn1 -- Temperature Source/RConn2
  Thermal Resistor/RConn1 -- Electrical Reference/LConn1 -- Controlled Current Source2/RConn2 -- Controlled Current Source/RConn2 -- Thermal Resistor2/RConn1 -- Controlled Current Source1/RConn2 -- Thermal Resistor1/RConn1
  Controlled Current Source/LConn1 -- Thermal Resistor2/LConn2
  Controlled Current Source1/LConn1 -- Thermal Resistor1/LConn2
  Controlled Current Source2/LConn1 -- Thermal Resistor/LConn2
  Simulink-PS Converter/RConn1 -- Controlled Current Source/RConn1
  Simulink-PS Converter1/RConn1 -- Controlled Current Source1/RConn1
  Controlled Current Source2/RConn1 -- Simulink-PS Converter2/RConn1
  ThRef1/LConn1 -- Controlled Heat Flow Rate Source/RConn2
  Simulink-PS Converter3/RConn1 -- Controlled Heat Flow Rate Source/RConn1
  Simulink-PS Converter4/RConn1 -- Controlled Heat Flow Rate Source1/RConn1
  ThRef2/LConn1 -- Controlled Heat Flow Rate Source1/RConn2
  ThRef3/LConn1 -- Controlled Heat Flow Rate Source2/RConn2
  Controlled Heat Flow Rate Source2/RConn1 -- Simulink-PS Converter5/RConn1
  Controlled Heat Flow Rate Source3/RConn1 -- Simulink-PS Converter6/RConn1
  ThRef4/LConn1 -- Controlled Heat Flow Rate Source3/RConn2

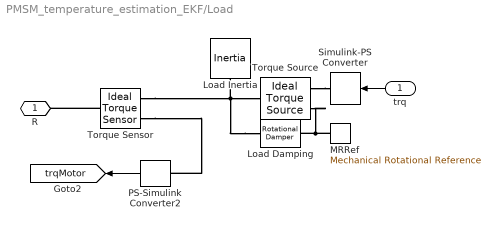
== system PMSM_temperature_estimation_EKF/Load ==
  trq : Inport
  Load Damping : fl_lib/Mechanical/Rotational Elements/Rotational Damper  D=30e3/(2*pi/60*2000)^2 N*m/(rad/s)  w_specify=off  w_priority=None  w=0 rad/s  w_nominal_specify=off  w_nominal_unit=rad/s  w_nominal_value=1  t_specify=off  t_priority=None  t=0 N*m  t_nominal_specify=off  t_nominal_unit=N*m  t_nominal_value=1
  Load Inertia : fl_lib/Mechanical/Rotational Elements/Inertia  inertia=1 kg*m^2  num_ports=foundation.enum.numPorts2.one  w_specify=off  w_priority=None  w=0 rad/s  w_nominal_specify=off  w_nominal_unit=rad/s  w_nominal_value=1  t_specify=off  t_priority=None  t=0 N*m  t_nominal_specify=off  t_nominal_unit=N*m  t_nominal_value=1
  MRRef : fl_lib/Mechanical/Rotational Elements/Mechanical Rotational Reference
  PS-Simulink Converter2 : nesl_utility/PS-Simulink Converter  PhysicalDomain=network_engine_domain  SubClassName=ps_output  LeftPortType=input  RightPortType=output  PseudoPeriodic=off  Frequencies=[]  VectorFormat=1-D array  Unit=N*m  AffineConversion=off
  Simulink-PS Converter : nesl_utility/Simulink-PS Converter  PhysicalDomain=network_engine_domain  SubClassName=ps_input  LeftPortType=input  RightPortType=output  PseudoPeriodic=off  Frequencies=[]  NoiseDistribution=none  NoiseParameters=[]  Unit=1  AffineConversion=off  FilteringAndDerivatives=zero  SimscapeFilterOrder=1  InputFilterTimeConstant=0.001  UdotUserProvided=1
  Torque Source : fl_lib/Mechanical/Mechanical Sources/Ideal Torque Source
  Torque Sensor : fl_lib/Mechanical/Mechanical Sensors/Ideal Torque Sensor
  R : PMIOPort  Side=Right
  tag scope: trqMotor=global
  wires:
  trq/1 -> Simulink-PS Converter/1
  PS-Simulink Converter2/1 -> [trqMotor]
  connections:
  Torque Source/RConn1 -- Simulink-PS Converter/RConn1
  MRRef/LConn1 -- Torque Source/RConn2 -- Load Damping/RConn1
  Load Damping/LConn1 -- Torque Sensor/RConn1 -- Load Inertia/LConn1 -- Torque Source/LConn1
  Torque Sensor/LConn1 -- R/RConn1
  Torque Sensor/RConn2 -- PS-Simulink Converter2/LConn1
